simulink model "untitled"  (R2015a)
settings: Solver=ode45  StartTime=0.0  StopTime=10.0  RelTol=1e-3
settings Model: Creator=saadc  LastModifiedBy=saadc

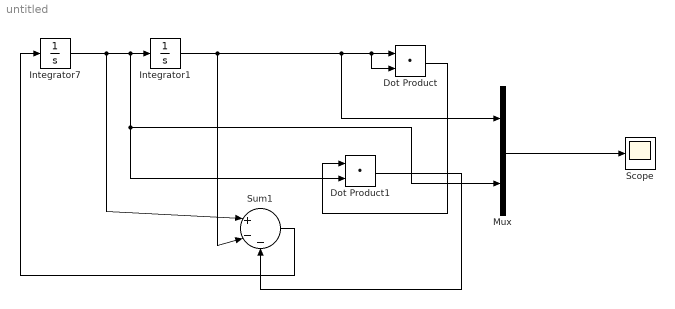
== system untitled ==
  Dot Product : DotProduct  InputSameDT=on  OutDataTypeStr=Inherit: Inherit via internal rule
  Dot Product1 : DotProduct  InputSameDT=on  OutDataTypeStr=Inherit: Inherit via internal rule
  Integrator1 : Integrator
  Integrator7 : Integrator
  Mux : Mux  Inputs=2
  Scope : Scope
  Sum1 : Sum  Inputs=|+--
  wires:
  Integrator7/1 -> Sum1/1, Mux/2, Dot Product1/2, Integrator1/1
  Integrator1/1 -> Sum1/2, Mux/1, Dot Product/2, Dot Product/1
  Dot Product/1 -> Dot Product1/1
  Sum1/1 -> Integrator7/1
  Mux/1 -> Scope/1
  Dot Product1/1 -> Sum1/3
